simulink model "siglearmV7XYZforcecontrol"  (R2024b)
settings: Solver=VariableStepAuto  StartTime=0.0  StopTime=0.6  RelTol=1e-3
undefined symbols (not defined in the file): X, Y, Z
libraries: sm_lib x40, nesl_utility x40
(part 1 of 2)
settings Model: Creator=ChangZhiYuan  LastModifiedBy=20844
settings OptimizationCC: ReuseModelBlockBuffer=off
settings RTWCC: GPUComputeCapability=3.5

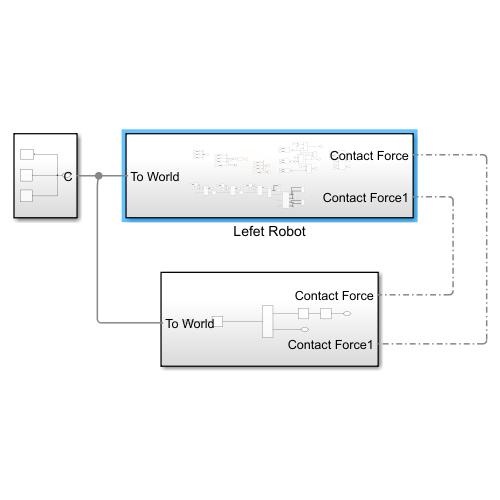
[thumbnail: Simulink's stored preview of the top-level diagram]
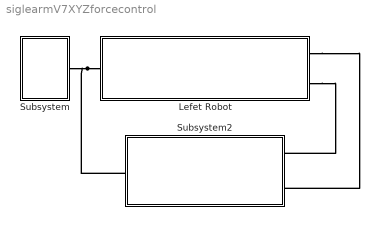
== system siglearmV7XYZforcecontrol ==
  Lefet Robot : Subsystem
  Subsystem : Subsystem
  Subsystem2 : Subsystem
  connections:
  Lefet Robot/LConn1 -- Subsystem2/LConn1 -- Subsystem/RConn1
  Lefet Robot/RConn2 -- Subsystem2/RConn1
  Lefet Robot/RConn1 -- Subsystem2/RConn2

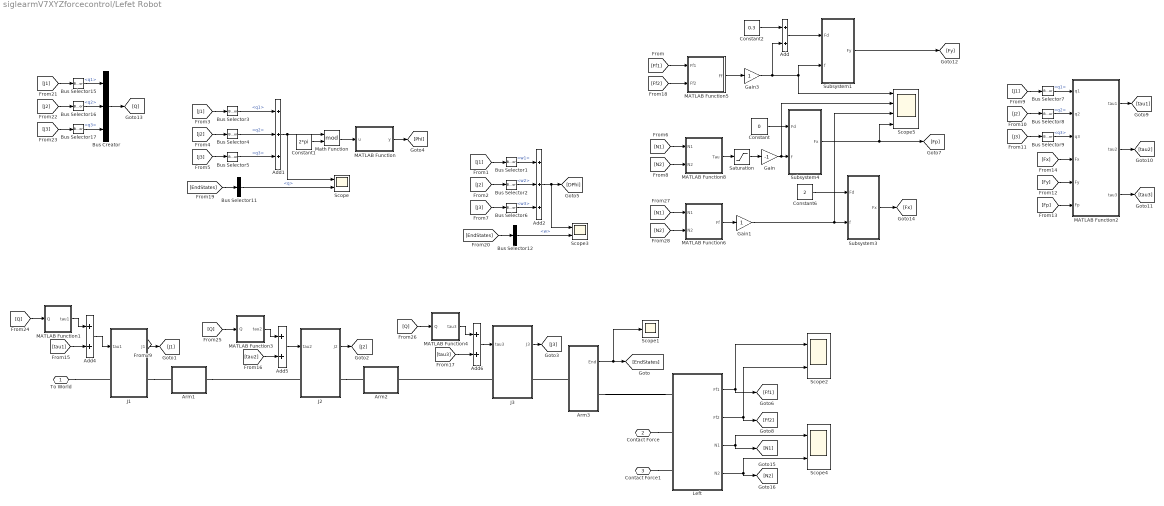
== system siglearmV7XYZforcecontrol/Lefet Robot ==
  Add{,4..6} (4 alike) : Sum
  Add1 : Sum  Inputs=+++
  Add2 : Sum  Inputs=+++
  Arm1 : Subsystem
  Arm2 : Subsystem
  Arm3 : Subsystem
  Bus Creator : BusCreator  Inputs=3
  Bus Selector1 : BusSelector  OutputSignals=w1
  Bus Selector11 : BusSelector  OutputSignals=q
  Bus Selector12 : BusSelector  OutputSignals=w
  Bus Selector15 : BusSelector  OutputSignals=q1
  Bus Selector16 : BusSelector  OutputSignals=q2
  Bus Selector17 : BusSelector  OutputSignals=q3
  Bus Selector2 : BusSelector  OutputSignals=w2
  Bus Selector3 : BusSelector  OutputSignals=q1
  Bus Selector4 : BusSelector  OutputSignals=q2
  Bus Selector5 : BusSelector  OutputSignals=q3
  Bus Selector6 : BusSelector  OutputSignals=w3
  Bus Selector7 : BusSelector  OutputSignals=q1
  Bus Selector8 : BusSelector  OutputSignals=q2
  Bus Selector9 : BusSelector  OutputSignals=q3
  Constant : Constant  Value=0
  Constant1 : Constant  Value=2*pi
  Constant2 : Constant  Value=0.3
  Constant6 : Constant  Value=2
  Gain : Gain  Gain=-1
  Gain1 : Gain
  Gain3 : Gain
  J1 : Subsystem
  J2 : Subsystem
  J3 : Subsystem
  Left : Subsystem
  MATLAB Function : MATLAB Function  TreatAsAtomicUnit=on
  MATLAB Function1 : MATLAB Function  TreatAsAtomicUnit=on
  MATLAB Function2 : MATLAB Function  TreatAsAtomicUnit=on
  MATLAB Function3 : MATLAB Function  TreatAsAtomicUnit=on
  MATLAB Function4 : MATLAB Function  TreatAsAtomicUnit=on
  MATLAB Function5 : MATLAB Function  TreatAsAtomicUnit=on
  MATLAB Function6 : MATLAB Function  TreatAsAtomicUnit=on
  MATLAB Function8 : MATLAB Function  TreatAsAtomicUnit=on
  Math Function : Math  Operator=mod
  Saturation : Saturate  UpperLimit=1  LowerLimit=-1
  Scope{,2..4} (4 alike) : Scope  NumInputPorts=2
  Scope1 : Scope
  Scope5 : Scope  NumInputPorts=4
  Subsystem1 : Subsystem
  Subsystem3 : Subsystem
  Subsystem4 : Subsystem
  To World : PMIOPort  Side=Left
  Contact Force : PMIOPort  Port=2  Side=Right
  Contact Force1 : PMIOPort  Port=3  Side=Right
  wires:
  Bus Selector9/1 -> MATLAB Function2/3(q3)  "<q3>"
  Add4/1 -> J1/1(tau1)
  Bus Selector7/1 -> MATLAB Function2/1(q1)  "<q1>"
  MATLAB Function2/1(tau1) -> [tau1]
  [EndStates] -> Bus Selector11/1
  [J2] -> Bus Selector4/1
  Bus Selector3/1 -> Add1/1  "<q1>"
  J2/1(J2) -> [J2]
  [J1] -> Bus Selector7/1
  [Fy] -> MATLAB Function2/5(Fy)
  Constant1/1 -> Math Function/2
  [J3] -> Bus Selector5/1
  Bus Selector2/1 -> Add2/2  "<w2>"
  [J1] -> Bus Selector1/1
  Bus Selector8/1 -> MATLAB Function2/2(q2)  "<q2>"
  Add1/1 -> Math Function/1, Scope/1
  Add6/1 -> J3/1(tau3)
  MATLAB Function2/2(tau2) -> [tau2]
  Math Function/1 -> MATLAB Function/1(u)
  Bus Selector12/1 -> Scope3/2  "<w>"
  [tau2] -> Add5/2
  Add2/1 -> Scope3/1, [DPhi]
  MATLAB Function2/3(tau3) -> [tau3]
  [J1] -> Bus Selector3/1
  [J3] -> Bus Selector9/1
  Bus Selector6/1 -> Add2/3  "<w3>"
  Bus Selector11/1 -> Scope/2  "<q>"
  [Fx] -> MATLAB Function2/4(Fx)
  Bus Selector4/1 -> Add1/2  "<q2>"
  Add5/1 -> J2/1(tau2)
  Bus Selector5/1 -> Add1/3  "<q3>"
  [J2] -> Bus Selector8/1
  J3/1(J3) -> [J3]
  J1/1(J1) -> [J1]
  [J3] -> Bus Selector6/1
  Bus Selector1/1 -> Add2/1  "<w1>"
  [EndStates] -> Bus Selector12/1
  [J2] -> Bus Selector2/1
  [Fp] -> MATLAB Function2/6(Fp)
  [tau1] -> Add4/2
  Subsystem4/1(Fx) -> Scope5/4, [Fp]
  Constant/1 -> Subsystem4/1(Fd)
  Arm3/1(End) -> Scope1/1, [EndStates]
  MATLAB Function/1(y) -> [Phi]
  Gain3/1 -> Add/2, Scope5/1, Subsystem1/2(f)
  [J2] -> Bus Selector16/1
  [J3] -> Bus Selector17/1
  [J1] -> Bus Selector15/1
  Bus Selector15/1 -> Bus Creator/1  "<q1>"
  Bus Selector16/1 -> Bus Creator/2  "<q2>"
  Bus Selector17/1 -> Bus Creator/3  "<q3>"
  Bus Creator/1 -> [Q]
  [Q] -> MATLAB Function1/1(Q)
  [Q] -> MATLAB Function3/1(Q)
  [tau3] -> Add6/2
  [Q] -> MATLAB Function4/1(Q)
  MATLAB Function1/1(tau1) -> Add4/1
  MATLAB Function3/1(tau2) -> Add5/1
  MATLAB Function4/1(tau3) -> Add6/1
  Constant6/1 -> Subsystem3/1(Fd)
  Subsystem3/1(Fx) -> [Fx]
  Subsystem1/1(Fy) -> [Fy]
  Constant2/1 -> Add/1
  Add/1 -> Subsystem1/1(Fd)
  Left/1(Ff1) -> [Ff1], Scope2/1
  Left/2(Ff2) -> [Ff2], Scope2/2
  Left/3(N1) -> [N1], Scope4/1
  Left/4(N2) -> [N2], Scope4/2
  [Ff1] -> MATLAB Function5/1(Ff1)
  [Ff2] -> MATLAB Function5/2(Ff2)
  MATLAB Function5/1(Ff) -> Gain3/1
  [N1] -> MATLAB Function6/1(N1)
  [N2] -> MATLAB Function6/2(N2)
  MATLAB Function6/1(Ff) -> Gain1/1
  Gain1/1 -> Scope5/3, Subsystem3/2(f)
  [N2] -> MATLAB Function8/2(N2)
  [N1] -> MATLAB Function8/1(N1)
  MATLAB Function8/1(Tau) -> Saturation/1
  Saturation/1 -> Gain/1
  Gain/1 -> Scope5/2, Subsystem4/2(f)
  connections:
  J1/RConn1 -- Arm1/LConn1
  Arm3/LConn1 -- J3/RConn1
  J3/LConn1 -- Arm2/RConn1
  J2/RConn1 -- Arm2/LConn1
  Left/LConn1 -- Arm3/RConn1
  Arm1/RConn1 -- J2/LConn1
  To World/RConn1 -- J1/LConn1
  Contact Force1/RConn1 -- Left/LConn3
  Contact Force/RConn1 -- Left/LConn2

== system siglearmV7XYZforcecontrol/Subsystem ==
  Mechanism Configuration : sm_lib/Utilities/Mechanism Configuration  UniformGravity=Constant  GravityVector=[0 -9.80665 0]  GravityVectorUnits=m/s^2  LinearizationDelta=0.001  JointModeTransitionNonlinearIterations=2
  Solver Configuration : nesl_utility/Solver Configuration  PhysicalDomain=network_engine_domain  SubClassName=solver  LeftPortType=input  RightPortType=generic  Tones=[]  Harmonics=[]  SimulateNoise=off  Profile=off  UseLocalSampling=off  EnableSwitchedLinearOptims=on  FrequencyDomain=off  UseCCode=off  RelTol=0.001  AbsTol=1e-06  MinStep=1e-09  ToWorkspace=off  RevertToSquareIcSolve=off  NumHomotopyIterations=100  PhasorMode=off  PhasorModeNumHarmonics=1  ConsistencySolver=NEWTON_FTOL  IndexReductionMethod=DerivativeReplacement  DoDC=off  ResidualTolerance=1e-09  ConsistencyTolSource=GLOBAL  ConsistencyAbsTol=0.001  ConsistencyRelTol=0.001  ConsistencyTolFactor=0.001  UseLocalSolver=off  LocalSolverChoice=NE_BACKWARD_EULER_ADVANCER  ResolveIndetEquations=on  FunctionEvalNumThread=1  LocalSolverSampleTime=0.001  DoFixedCost=off  MaxNonlinIter=3  MaxModeIter=2  ComputeImpulses=off  ImpulseIterations=2  LinearAlgebra=auto  LinearAlgebraNumThread=0  EquationFormulation=NE_TIME_EF  DelaysMemoryBudget=1024  AutomaticFiltering=on  FilteringTimeConstant=0.001  PartitionStorageMethod=AS_NEEDED  PartitionMemoryBudget=1024  PartitionMethod=ROBUST  MultibodyUseLocalSolver=off  MultibodyLocalSolverChoice=ODE1  MultibodyLocalSolverSampleTime=0.001
  World Frame : sm_lib/Frames and Transforms/World Frame
  C : PMIOPort  Side=Right
  connections:
  C/RConn1 -- Mechanism Configuration/RConn1 -- World Frame/RConn1 -- Solver Configuration/RConn1

== system siglearmV7XYZforcecontrol/Subsystem2 ==
  Object : sm_lib/Body Elements/Brick Solid  BrickDimensions=[0.01 1.5 0.5]  BrickDimensionsUnits=m  ExportEntireGeometry=on  InertiaType=CalculateFromGeometry  BasedOnType=Density  Density=100  DensityUnits=kg/m^3  Mass=1  MassUnits=kg  CenterOfMass=[0 0 0]  CenterOfMassUnits=m  MomentsOfInertia=[1 1 1]  MomentsOfInertiaUnits=kg*m^2  ProductsOfInertia=[0 0 0]  ProductsOfInertiaUnits=kg*m^2  GraphicType=FromGeometry  MarkerShape=Sphere  MarkerSize=10  GraphicVisPropType=SimpleVisualProperties  GraphicDiffuseColor=[0.5 0.5 0.5]  GraphicOpacity=1.0  GraphicSpecularColor=[0.5 0.5 0.5 1.0]  GraphicAmbientColor=[0.15 0.15 0.15 1.0]  GraphicEmissiveColor=[0.0 0.0 0.0 1.0]  GraphicShininess=75  DoExposeReferenceFrame=on  SerializedFrames=<Frames><Frame><Id>Frame1</Id><Value><Name>F1</Name><Origin><Source>GeometricFeature</Source><FeatureName>-x surface</FeatureName></Origin><PrimaryAxis><DefinedDirection>+Z</DefinedDirection><Source>ReferenceFrame</Source><SourceDirection>+Z</SourceDirection><FeatureName></FeatureName></PrimaryAxis><SecondaryAxis><DefinedDirection>+X</DefinedDirection><Source>ReferenceFrame</Source><SourceDirection>+X</SourceDirection><FeatureName></FeatureName></SecondaryAxis></Value></Frame></Frames>
  Revolved Solid : sm_lib/Body Elements/Revolved Solid  RevolutionCrossSection=[1 0.1; 1 -0.1; 1.01 -0.1; 1.01 0.1]  RevolutionCrossSectionUnits=m  RevolutionExtent=Custom  RevolutionAngle=30  RevolutionAngleUnits=deg  ExportConvexHullGeometry=on  InertiaType=CalculateFromGeometry  BasedOnType=Density  Density=1000  DensityUnits=kg/m^3  Mass=1  MassUnits=kg  CenterOfMass=[0 0 0]  CenterOfMassUnits=m  MomentsOfInertia=[1 1 1]  MomentsOfInertiaUnits=kg*m^2  ProductsOfInertia=[0 0 0]  ProductsOfInertiaUnits=kg*m^2  GraphicType=FromGeometry  MarkerShape=Sphere  MarkerSize=10  GraphicVisPropType=SimpleVisualProperties  GraphicDiffuseColor=[0.5 0.5 0.5]  GraphicOpacity=1.0  GraphicSpecularColor=[0.5 0.5 0.5 1.0]  GraphicAmbientColor=[0.15 0.15 0.15 1.0]  GraphicEmissiveColor=[0.0 0.0 0.0 1.0]  GraphicShininess=75  DoExposeReferenceFrame=on  SerializedFrames=<Frames/>
  Rigid Transform : sm_lib/Frames and Transforms/Rigid Transform  RotationMethod=None  FollAlignAxisA=+X  BaseAlignAxisA=+Y  FollAlignAxisB=+Y  BaseAlignAxisB=+Z  RotationStandardAxis=+Z  RotationAngle=0.0  RotationAngleUnits=deg  RotationArbitraryAxis=[0 0 1]  RotationSequenceAxes=FollowerAxes  RotationSequence=XYX  RotationSequenceAngles=[0 0 0]  RotationSequenceAnglesUnits=deg  RotationMatrix=[1 0 0; 0 1 0; 0 0 1]  Quaternion=[1 0 0 0]  TranslationMethod=Cartesian  TranslationCartesianOffset=[0.4505+0.005 0.5 0]  TranslationCartesianOffsetUnits=m  TranslationStandardAxis=+Z  TranslationStandardOffset=0  TranslationStandardOffsetUnits=m  TranslationROffset=0  TranslationROffsetUnits=m  TranslationThetaOffset=0  TranslationThetaOffsetUnits=deg  TranslationZOffset=0  TranslationZOffsetUnits=m
  Rigid Transform1 : sm_lib/Frames and Transforms/Rigid Transform  RotationMethod=StandardAxis  FollAlignAxisA=+X  BaseAlignAxisA=+Y  FollAlignAxisB=+Y  BaseAlignAxisB=+Z  RotationStandardAxis=+Z  RotationAngle=180  RotationAngleUnits=deg  RotationArbitraryAxis=[0 0 1]  RotationSequenceAxes=FollowerAxes  RotationSequence=XYX  RotationSequenceAngles=[0 0 0]  RotationSequenceAnglesUnits=deg  RotationMatrix=[1 0 0; 0 1 0; 0 0 1]  Quaternion=[1 0 0 0]  TranslationMethod=Cartesian  TranslationCartesianOffset=[0.98 0.1 0]  TranslationCartesianOffsetUnits=m  TranslationStandardAxis=+X  TranslationStandardOffset=0.98  TranslationStandardOffsetUnits=m  TranslationROffset=0  TranslationROffsetUnits=m  TranslationThetaOffset=0  TranslationThetaOffsetUnits=deg  TranslationZOffset=0  TranslationZOffsetUnits=m
  To World : PMIOPort  Side=Left
  Contact Force : PMIOPort  Port=2  Side=Right
  Contact Force1 : PMIOPort  Port=3  Side=Right
  connections:
  Rigid Transform/RConn1 -- Object/RConn1
  Rigid Transform/LConn1 -- To World/RConn1
  Object/LConn2 -- Contact Force/RConn1
  Rigid Transform1/LConn1 -- Object/LConn1
  Revolved Solid/RConn1 -- Rigid Transform1/RConn1
  Contact Force1/RConn1 -- Revolved Solid/LConn1

== system siglearmV7XYZforcecontrol/Lefet Robot/Arm1 ==
  Brick Solid : sm_lib/Body Elements/Brick Solid  BrickDimensions=[0.5 0.05 0.05]  BrickDimensionsUnits=m  ExportEntireGeometry=off  InertiaType=CalculateFromGeometry  BasedOnType=Density  Density=100  DensityUnits=kg/m^3  Mass=1  MassUnits=kg  CenterOfMass=[0 0 0]  CenterOfMassUnits=m  MomentsOfInertia=[1 1 1]  MomentsOfInertiaUnits=kg*m^2  ProductsOfInertia=[0 0 0]  ProductsOfInertiaUnits=kg*m^2  GraphicType=FromGeometry  MarkerShape=Sphere  MarkerSize=10  GraphicVisPropType=SimpleVisualProperties  GraphicDiffuseColor=[0.0 1.0 0.2]  GraphicOpacity=1.0  GraphicSpecularColor=[0.5 0.5 0.5 1.0]  GraphicAmbientColor=[0.15 0.15 0.15 1.0]  GraphicEmissiveColor=[0.0 0.0 0.0 1.0]  GraphicShininess=75  DoExposeReferenceFrame=on  SerializedFrames=<Frames><Frame><Id>Frame1</Id><Value><Name>F</Name><Origin><Source>CenterOfMassFrame</Source><FeatureName></FeatureName></Origin><PrimaryAxis><DefinedDirection>+Z</DefinedDirection><Source>ReferenceFrame</Source><SourceDirection>+Z</SourceDirection><FeatureName></FeatureName></PrimaryAxis><SecondaryAxis><DefinedDirection>+X</DefinedDirection><Source>ReferenceFrame</Source><SourceDirection>+X</SourceDirection><FeatureName></FeatureName></SecondaryAxis></Value></Frame></Frames>
  Cylindrical Solid : sm_lib/Body Elements/Cylindrical Solid  CylinderRadius=0.04  CylinderRadiusUnits=m  CylinderLength=0.06  CylinderLengthUnits=m  ExportEntireGeometry=off  InertiaType=CalculateFromGeometry  BasedOnType=Density  Density=1e-6  DensityUnits=kg/m^3  Mass=1  MassUnits=kg  CenterOfMass=[0 0 0]  CenterOfMassUnits=m  MomentsOfInertia=[1 1 1]  MomentsOfInertiaUnits=kg*m^2  ProductsOfInertia=[0 0 0]  ProductsOfInertiaUnits=kg*m^2  GraphicType=FromGeometry  MarkerShape=Sphere  MarkerSize=10  GraphicVisPropType=SimpleVisualProperties  GraphicDiffuseColor=[1.0 0.0 0.2]  GraphicOpacity=1.0  GraphicSpecularColor=[0.5 0.5 0.5 1.0]  GraphicAmbientColor=[0.15 0.15 0.15 1.0]  GraphicEmissiveColor=[0.0 0.0 0.0 1.0]  GraphicShininess=75  DoExposeReferenceFrame=on  SerializedFrames=<Frames><Frame><Id>Frame1</Id><Value><Name>F1</Name><Origin><Source>CenterOfMassFrame</Source><FeatureName></FeatureName></Origin><PrimaryAxis><DefinedDirection>+Z</DefinedDirection><Source>ReferenceFrame</Source><SourceDirection>+Z</SourceDirection><FeatureName></FeatureName></PrimaryAxis><SecondaryAxis><DefinedDirection>+X</DefinedDirection><Source>ReferenceFrame</Source><SourceDirection>+X</SourceDirection><FeatureName></FeatureName></SecondaryAxis></Value></Frame></Frames>
  Rigid Transform : sm_lib/Frames and Transforms/Rigid Transform  RotationMethod=None  FollAlignAxisA=+X  BaseAlignAxisA=+Y  FollAlignAxisB=+Y  BaseAlignAxisB=+Z  RotationStandardAxis=+Z  RotationAngle=0.0  RotationAngleUnits=deg  RotationArbitraryAxis=[0 0 1]  RotationSequenceAxes=FollowerAxes  RotationSequence=XYX  RotationSequenceAngles=[0 0 0]  RotationSequenceAnglesUnits=deg  RotationMatrix=[1 0 0; 0 1 0; 0 0 1]  Quaternion=[1 0 0 0]  TranslationMethod=StandardAxis  TranslationCartesianOffset=[0 0 0]  TranslationCartesianOffsetUnits=m  TranslationStandardAxis=+X  TranslationStandardOffset=0.25  TranslationStandardOffsetUnits=m  TranslationROffset=0  TranslationROffsetUnits=m  TranslationThetaOffset=0  TranslationThetaOffsetUnits=deg  TranslationZOffset=0  TranslationZOffsetUnits=m
  Rigid Transform1 : sm_lib/Frames and Transforms/Rigid Transform  RotationMethod=None  FollAlignAxisA=+X  BaseAlignAxisA=+Y  FollAlignAxisB=+Y  BaseAlignAxisB=+Z  RotationStandardAxis=+Z  RotationAngle=0.0  RotationAngleUnits=deg  RotationArbitraryAxis=[0 0 1]  RotationSequenceAxes=FollowerAxes  RotationSequence=XYX  RotationSequenceAngles=[0 0 0]  RotationSequenceAnglesUnits=deg  RotationMatrix=[1 0 0; 0 1 0; 0 0 1]  Quaternion=[1 0 0 0]  TranslationMethod=StandardAxis  TranslationCartesianOffset=[0 0 0]  TranslationCartesianOffsetUnits=m  TranslationStandardAxis=+X  TranslationStandardOffset=0.25  TranslationStandardOffsetUnits=m  TranslationROffset=0  TranslationROffsetUnits=m  TranslationThetaOffset=0  TranslationThetaOffsetUnits=deg  TranslationZOffset=0  TranslationZOffsetUnits=m
  To J1 : PMIOPort  Side=Left
  To J2 : PMIOPort  Port=2  Side=Right
  connections:
  Brick Solid/LConn1 -- Rigid Transform1/LConn1
  Rigid Transform/RConn1 -- Brick Solid/RConn1
  To J2/RConn1 -- Rigid Transform1/RConn1
  Cylindrical Solid/RConn1 -- To J1/RConn1
  Cylindrical Solid/LConn1 -- Rigid Transform/LConn1

== system siglearmV7XYZforcecontrol/Lefet Robot/Arm2 ==
  Brick Solid1 : sm_lib/Body Elements/Brick Solid  BrickDimensions=[0.5 0.05 0.05]  BrickDimensionsUnits=m  ExportEntireGeometry=off  InertiaType=CalculateFromGeometry  BasedOnType=Density  Density=100  DensityUnits=kg/m^3  Mass=1  MassUnits=kg  CenterOfMass=[0 0 0]  CenterOfMassUnits=m  MomentsOfInertia=[1 1 1]  MomentsOfInertiaUnits=kg*m^2  ProductsOfInertia=[0 0 0]  ProductsOfInertiaUnits=kg*m^2  GraphicType=FromGeometry  MarkerShape=Sphere  MarkerSize=10  GraphicVisPropType=SimpleVisualProperties  GraphicDiffuseColor=[0.2 1.0 0.0]  GraphicOpacity=1.0  GraphicSpecularColor=[0.5 0.5 0.5 1.0]  GraphicAmbientColor=[0.15 0.15 0.15 1.0]  GraphicEmissiveColor=[0.0 0.0 0.0 1.0]  GraphicShininess=75  DoExposeReferenceFrame=on  SerializedFrames=<Frames><Frame><Id>Frame1</Id><Value><Name>F</Name><Origin><Source>CenterOfMassFrame</Source><FeatureName></FeatureName></Origin><PrimaryAxis><DefinedDirection>+Z</DefinedDirection><Source>ReferenceFrame</Source><SourceDirection>+Z</SourceDirection><FeatureName></FeatureName></PrimaryAxis><SecondaryAxis><DefinedDirection>+X</DefinedDirection><Source>ReferenceFrame</Source><SourceDirection>+X</SourceDirection><FeatureName></FeatureName></SecondaryAxis></Value></Frame></Frames>
  Cylindrical Solid : sm_lib/Body Elements/Cylindrical Solid  CylinderRadius=0.04  CylinderRadiusUnits=m  CylinderLength=0.06  CylinderLengthUnits=m  ExportEntireGeometry=off  InertiaType=CalculateFromGeometry  BasedOnType=Density  Density=1e-6  DensityUnits=kg/m^3  Mass=1  MassUnits=kg  CenterOfMass=[0 0 0]  CenterOfMassUnits=m  MomentsOfInertia=[1 1 1]  MomentsOfInertiaUnits=kg*m^2  ProductsOfInertia=[0 0 0]  ProductsOfInertiaUnits=kg*m^2  GraphicType=FromGeometry  MarkerShape=Sphere  MarkerSize=10  GraphicVisPropType=SimpleVisualProperties  GraphicDiffuseColor=[1.0 0.0 0.2]  GraphicOpacity=1.0  GraphicSpecularColor=[0.5 0.5 0.5 1.0]  GraphicAmbientColor=[0.15 0.15 0.15 1.0]  GraphicEmissiveColor=[0.0 0.0 0.0 1.0]  GraphicShininess=75  DoExposeReferenceFrame=on  SerializedFrames=<Frames><Frame><Id>Frame1</Id><Value><Name>F1</Name><Origin><Source>CenterOfMassFrame</Source><FeatureName></FeatureName></Origin><PrimaryAxis><DefinedDirection>+Z</DefinedDirection><Source>ReferenceFrame</Source><SourceDirection>+Z</SourceDirection><FeatureName></FeatureName></PrimaryAxis><SecondaryAxis><DefinedDirection>+X</DefinedDirection><Source>ReferenceFrame</Source><SourceDirection>+X</SourceDirection><FeatureName></FeatureName></SecondaryAxis></Value></Frame></Frames>
  Rigid Transform2 : sm_lib/Frames and Transforms/Rigid Transform  RotationMethod=None  FollAlignAxisA=+X  BaseAlignAxisA=+Y  FollAlignAxisB=+Y  BaseAlignAxisB=+Z  RotationStandardAxis=+Z  RotationAngle=0.0  RotationAngleUnits=deg  RotationArbitraryAxis=[0 0 1]  RotationSequenceAxes=FollowerAxes  RotationSequence=XYX  RotationSequenceAngles=[0 0 0]  RotationSequenceAnglesUnits=deg  RotationMatrix=[1 0 0; 0 1 0; 0 0 1]  Quaternion=[1 0 0 0]  TranslationMethod=StandardAxis  TranslationCartesianOffset=[0 0 0]  TranslationCartesianOffsetUnits=m  TranslationStandardAxis=+X  TranslationStandardOffset=0.25  TranslationStandardOffsetUnits=m  TranslationROffset=0  TranslationROffsetUnits=m  TranslationThetaOffset=0  TranslationThetaOffsetUnits=deg  TranslationZOffset=0  TranslationZOffsetUnits=m
  Rigid Transform3 : sm_lib/Frames and Transforms/Rigid Transform  RotationMethod=None  FollAlignAxisA=+X  BaseAlignAxisA=+Y  FollAlignAxisB=+Y  BaseAlignAxisB=+Z  RotationStandardAxis=+Z  RotationAngle=0.0  RotationAngleUnits=deg  RotationArbitraryAxis=[0 0 1]  RotationSequenceAxes=FollowerAxes  RotationSequence=XYX  RotationSequenceAngles=[0 0 0]  RotationSequenceAnglesUnits=deg  RotationMatrix=[1 0 0; 0 1 0; 0 0 1]  Quaternion=[1 0 0 0]  TranslationMethod=StandardAxis  TranslationCartesianOffset=[0 0 0]  TranslationCartesianOffsetUnits=m  TranslationStandardAxis=+X  TranslationStandardOffset=0.25  TranslationStandardOffsetUnits=m  TranslationROffset=0  TranslationROffsetUnits=m  TranslationThetaOffset=0  TranslationThetaOffsetUnits=deg  TranslationZOffset=0  TranslationZOffsetUnits=m
  To J2 : PMIOPort  Side=Left
  To J3 : PMIOPort  Port=2  Side=Right
  connections:
  Rigid Transform2/RConn1 -- Brick Solid1/RConn1
  To J3/RConn1 -- Rigid Transform3/RConn1
  Brick Solid1/LConn1 -- Rigid Transform3/LConn1
  Cylindrical Solid/RConn1 -- To J2/RConn1
  Cylindrical Solid/LConn1 -- Rigid Transform2/LConn1

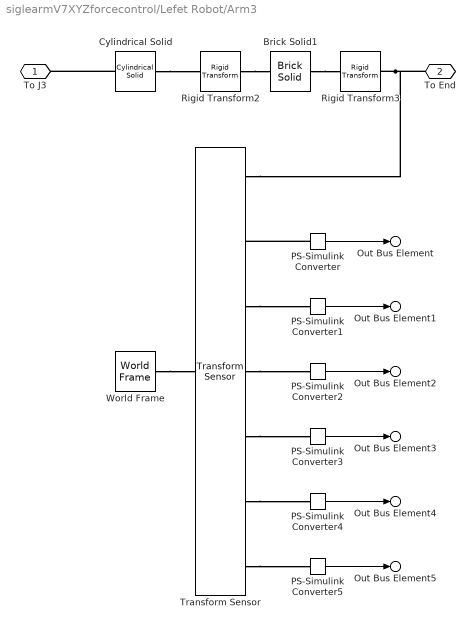
== system siglearmV7XYZforcecontrol/Lefet Robot/Arm3 ==
  Brick Solid1 : sm_lib/Body Elements/Brick Solid  BrickDimensions=[0.1 0.03 0.03]  BrickDimensionsUnits=m  ExportEntireGeometry=off  InertiaType=CalculateFromGeometry  BasedOnType=Density  Density=100  DensityUnits=kg/m^3  Mass=1  MassUnits=kg  CenterOfMass=[0 0 0]  CenterOfMassUnits=m  MomentsOfInertia=[1 1 1]  MomentsOfInertiaUnits=kg*m^2  ProductsOfInertia=[0 0 0]  ProductsOfInertiaUnits=kg*m^2  GraphicType=FromGeometry  MarkerShape=Sphere  MarkerSize=10  GraphicVisPropType=SimpleVisualProperties  GraphicDiffuseColor=[0.2 1.0 0.0]  GraphicOpacity=1.0  GraphicSpecularColor=[0.5 0.5 0.5 1.0]  GraphicAmbientColor=[0.15 0.15 0.15 1.0]  GraphicEmissiveColor=[0.0 0.0 0.0 1.0]  GraphicShininess=75  DoExposeReferenceFrame=on  SerializedFrames=<Frames><Frame><Id>Frame1</Id><Value><Name>F</Name><Origin><Source>CenterOfMassFrame</Source><FeatureName></FeatureName></Origin><PrimaryAxis><DefinedDirection>+Z</DefinedDirection><Source>ReferenceFrame</Source><SourceDirection>+Z</SourceDirection><FeatureName></FeatureName></PrimaryAxis><SecondaryAxis><DefinedDirection>+X</DefinedDirection><Source>ReferenceFrame</Source><SourceDirection>+X</SourceDirection><FeatureName></FeatureName></SecondaryAxis></Value></Frame></Frames>
  Cylindrical Solid : sm_lib/Body Elements/Cylindrical Solid  CylinderRadius=0.04  CylinderRadiusUnits=m  CylinderLength=0.06  CylinderLengthUnits=m  ExportEntireGeometry=off  InertiaType=CalculateFromGeometry  BasedOnType=Density  Density=1e-6  DensityUnits=kg/m^3  Mass=1  MassUnits=kg  CenterOfMass=[0 0 0]  CenterOfMassUnits=m  MomentsOfInertia=[1 1 1]  MomentsOfInertiaUnits=kg*m^2  ProductsOfInertia=[0 0 0]  ProductsOfInertiaUnits=kg*m^2  GraphicType=FromGeometry  MarkerShape=Sphere  MarkerSize=10  GraphicVisPropType=SimpleVisualProperties  GraphicDiffuseColor=[1.0 0.0 0.2]  GraphicOpacity=1.0  GraphicSpecularColor=[0.5 0.5 0.5 1.0]  GraphicAmbientColor=[0.15 0.15 0.15 1.0]  GraphicEmissiveColor=[0.0 0.0 0.0 1.0]  GraphicShininess=75  DoExposeReferenceFrame=on  SerializedFrames=<Frames><Frame><Id>Frame1</Id><Value><Name>F1</Name><Origin><Source>CenterOfMassFrame</Source><FeatureName></FeatureName></Origin><PrimaryAxis><DefinedDirection>+Z</DefinedDirection><Source>ReferenceFrame</Source><SourceDirection>+Z</SourceDirection><FeatureName></FeatureName></PrimaryAxis><SecondaryAxis><DefinedDirection>+X</DefinedDirection><Source>ReferenceFrame</Source><SourceDirection>+X</SourceDirection><FeatureName></FeatureName></SecondaryAxis></Value></Frame></Frames>
  PS-Simulink Converter{,1..5} (6 alike) : nesl_utility/PS-Simulink Converter  PhysicalDomain=network_engine_domain  SubClassName=ps_output  LeftPortType=input  RightPortType=output  PseudoPeriodic=off  Frequencies=[]  VectorFormat=inherit  Unit=inherit  AffineConversion=off
  Rigid Transform2 : sm_lib/Frames and Transforms/Rigid Transform  RotationMethod=None  FollAlignAxisA=+X  BaseAlignAxisA=+Y  FollAlignAxisB=+Y  BaseAlignAxisB=+Z  RotationStandardAxis=+Z  RotationAngle=0.0  RotationAngleUnits=deg  RotationArbitraryAxis=[0 0 1]  RotationSequenceAxes=FollowerAxes  RotationSequence=XYX  RotationSequenceAngles=[0 0 0]  RotationSequenceAnglesUnits=deg  RotationMatrix=[1 0 0; 0 1 0; 0 0 1]  Quaternion=[1 0 0 0]  TranslationMethod=StandardAxis  TranslationCartesianOffset=[0 0 0]  TranslationCartesianOffsetUnits=m  TranslationStandardAxis=+X  TranslationStandardOffset=0.05  TranslationStandardOffsetUnits=m  TranslationROffset=0  TranslationROffsetUnits=m  TranslationThetaOffset=0  TranslationThetaOffsetUnits=deg  TranslationZOffset=0  TranslationZOffsetUnits=m
  Rigid Transform3 : sm_lib/Frames and Transforms/Rigid Transform  RotationMethod=None  FollAlignAxisA=+X  BaseAlignAxisA=+Y  FollAlignAxisB=+Y  BaseAlignAxisB=+Z  RotationStandardAxis=+Z  RotationAngle=0.0  RotationAngleUnits=deg  RotationArbitraryAxis=[0 0 1]  RotationSequenceAxes=FollowerAxes  RotationSequence=XYX  RotationSequenceAngles=[0 0 0]  RotationSequenceAnglesUnits=deg  RotationMatrix=[1 0 0; 0 1 0; 0 0 1]  Quaternion=[1 0 0 0]  TranslationMethod=StandardAxis  TranslationCartesianOffset=[0 0 0]  TranslationCartesianOffsetUnits=m  TranslationStandardAxis=+X  TranslationStandardOffset=0.05  TranslationStandardOffsetUnits=m  TranslationROffset=0  TranslationROffsetUnits=m  TranslationThetaOffset=0  TranslationThetaOffsetUnits=deg  TranslationZOffset=0  TranslationZOffsetUnits=m
  Transform Sensor : sm_lib/Frames and Transforms/Transform Sensor  MeasurementFrame=World  RotationSequence=XYX  SenseAngle=on  SenseAxis=off  SenseQ=off  SenseR=off  SenseRotationSequence=off  SenseOmegaX=off  SenseOmegaY=off  SenseOmegaZ=on  SenseOmega=off  SenseQDot=off  SenseRDot=off  SenseRotationSequenceDot=off  SenseAlphaX=off  SenseAlphaY=off  SenseAlphaZ=off  SenseAlpha=off  SenseQDDot=off  SenseRDDot=off  SenseX=on  SenseY=on  SenseZ=off  SenseXYZ=off  SenseRad=off  SenseAzim=off  SenseDist=off  SenseInc=off  SenseXDot=on  SenseYDot=on  SenseZDot=off  SenseXYZDot=off  SenseRadDot=off  SenseAzimDot=off  SenseDistDot=off  SenseIncDot=off  SenseXDDot=off  SenseYDDot=off  SenseZDDot=off  SenseXYZDDot=off  SenseRadDDot=off  SenseAzimDDot=off  SenseDistDDot=off  SenseIncDDot=off
  World Frame : sm_lib/Frames and Transforms/World Frame
  To J3 : PMIOPort  Side=Left
  To End : PMIOPort  Port=2  Side=Right
  Out Bus Element : Outport  PortName=End  Element=q
  Out Bus Element1 : Outport  PortName=End  Element=w
  Out Bus Element2 : Outport  PortName=End  Element=x
  Out Bus Element3 : Outport  PortName=End  Element=y
  Out Bus Element4 : Outport  PortName=End  Element=vx
  Out Bus Element5 : Outport  PortName=End  Element=vy
  wires:
  PS-Simulink Converter/1 -> Out Bus Element/1
  PS-Simulink Converter1/1 -> Out Bus Element1/1
  PS-Simulink Converter2/1 -> Out Bus Element2/1
  PS-Simulink Converter5/1 -> Out Bus Element5/1
  PS-Simulink Converter4/1 -> Out Bus Element4/1
  PS-Simulink Converter3/1 -> Out Bus Element3/1
  connections:
  Rigid Transform2/RConn1 -- Brick Solid1/RConn1
  Rigid Transform3/RConn1 -- To End/RConn1 -- Transform Sensor/RConn1
  Brick Solid1/LConn1 -- Rigid Transform3/LConn1
  Cylindrical Solid/RConn1 -- To J3/RConn1
  Cylindrical Solid/LConn1 -- Rigid Transform2/LConn1
  World Frame/RConn1 -- Transform Sensor/LConn1
  PS-Simulink Converter/LConn1 -- Transform Sensor/RConn2
  Transform Sensor/RConn3 -- PS-Simulink Converter1/LConn1
  Transform Sensor/RConn5 -- PS-Simulink Converter3/LConn1
  Transform Sensor/RConn4 -- PS-Simulink Converter2/LConn1
  Transform Sensor/RConn7 -- PS-Simulink Converter5/LConn1
  Transform Sensor/RConn6 -- PS-Simulink Converter4/LConn1

== system siglearmV7XYZforcecontrol/Lefet Robot/J1 ==
  tau1 : Inport
  Constant : Constant  Value=2*pi
  Math Function : Math  Operator=mod
  PS-Simulink Converter4 : nesl_utility/PS-Simulink Converter  PhysicalDomain=network_engine_domain  SubClassName=ps_output  LeftPortType=input  RightPortType=output  PseudoPeriodic=off  Frequencies=[]  VectorFormat=inherit  Unit=inherit  AffineConversion=off
  PS-Simulink Converter5 : nesl_utility/PS-Simulink Converter  PhysicalDomain=network_engine_domain  SubClassName=ps_output  LeftPortType=input  RightPortType=output  PseudoPeriodic=off  Frequencies=[]  VectorFormat=inherit  Unit=inherit  AffineConversion=off
  Revolute Joint3 : sm_lib/Joints/Revolute Joint  JointMode=Normal  CompositeWrenchDir=FollowerOnBase  CompositeWrenchFrame=BaseFrame  SenseConstraintForce=off  SenseConstraintTorque=off  SenseTotalForce=off  SenseTotalTorque=off  PositionTargetSpecify=on  PositionTargetPriority=High  PositionTargetValue=1.7464  PositionTargetValueUnits=rad  VelocityTargetSpecify=off  VelocityTargetPriority=High  VelocityTargetValue=0  VelocityTargetValueUnits=deg/s  EquilibriumPosition=0  EquilibriumPositionUnits=deg  SpringStiffness=0  SpringStiffnessUnits=N*m/deg  DampingCoefficient=0  DampingCoefficientUnits=N*m/(deg/s)  LowerLimitSpecify=off  LowerLimitBound=-90  LowerLimitBoundUnits=deg  LowerLimitStiffness=1e4  LowerLimitStiffnessUnits=N*m/deg  LowerLimitDamping=10  LowerLimitDampingUnits=N*m/(deg/s)  LowerLimitTransitionRegionWidth=0.1  LowerLimitTransitionRegionWidthUnits=deg  UpperLimitSpecify=off  UpperLimitBound=90  UpperLimitBoundUnits=deg  UpperLimitStiffness=1e4  UpperLimitStiffnessUnits=N*m/deg  UpperLimitDamping=10  UpperLimitDampingUnits=N*m/(deg/s)  UpperLimitTransitionRegionWidth=0.1  UpperLimitTransitionRegionWidthUnits=deg  TorqueActuationMode=InputTorque  MotionActuationMode=ComputedMotion  SensePosition=on  SenseVelocity=on  SenseAcceleration=off  SenseTorqueForce=off  SenseLowerLimitTorqueForce=off  SenseUpperLimitTorqueForce=off
  Simulink-PS Converter : nesl_utility/Simulink-PS Converter  PhysicalDomain=network_engine_domain  SubClassName=ps_input  LeftPortType=input  RightPortType=output  PseudoPeriodic=off  Frequencies=[]  NoiseDistribution=none  NoiseParameters=[]  Unit=1  AffineConversion=off  FilteringAndDerivatives=provide  SimscapeFilterOrder=1  InputFilterTimeConstant=0.001  UdotUserProvided=0
  Conn1 : PMIOPort  Side=Right
  Conn2 : PMIOPort  Port=2  Side=Left
  Bus Element Out : Outport  PortName=J1  Element=q1
  Bus Element Out1 : Outport  PortName=J1  Element=w1
  wires:
  tau1/1 -> Simulink-PS Converter/1
  PS-Simulink Converter5/1 -> Bus Element Out1/1
  PS-Simulink Converter4/1 -> Bus Element Out/1, Math Function/1
  Constant/1 -> Math Function/2
  connections:
  Revolute Joint3/LConn2 -- Simulink-PS Converter/RConn1
  Revolute Joint3/RConn2 -- PS-Simulink Converter4/LConn1
  Revolute Joint3/RConn3 -- PS-Simulink Converter5/LConn1
  Revolute Joint3/RConn1 -- Conn1/RConn1
  Conn2/RConn1 -- Revolute Joint3/LConn1

== system siglearmV7XYZforcecontrol/Lefet Robot/J2 ==
  tau2 : Inport
  Constant : Constant  Value=2*pi
  Math Function : Math  Operator=mod
  PS-Simulink Converter2 : nesl_utility/PS-Simulink Converter  PhysicalDomain=network_engine_domain  SubClassName=ps_output  LeftPortType=input  RightPortType=output  PseudoPeriodic=off  Frequencies=[]  VectorFormat=inherit  Unit=inherit  AffineConversion=off
  PS-Simulink Converter3 : nesl_utility/PS-Simulink Converter  PhysicalDomain=network_engine_domain  SubClassName=ps_output  LeftPortType=input  RightPortType=output  PseudoPeriodic=off  Frequencies=[]  VectorFormat=inherit  Unit=inherit  AffineConversion=off
  Revolute Joint1 : sm_lib/Joints/Revolute Joint  JointMode=Normal  CompositeWrenchDir=FollowerOnBase  CompositeWrenchFrame=BaseFrame  SenseConstraintForce=off  SenseConstraintTorque=off  SenseTotalForce=off  SenseTotalTorque=off  PositionTargetSpecify=on  PositionTargetPriority=High  PositionTargetValue=-2.2523  PositionTargetValueUnits=rad  VelocityTargetSpecify=off  VelocityTargetPriority=High  VelocityTargetValue=0  VelocityTargetValueUnits=deg/s  EquilibriumPosition=0  EquilibriumPositionUnits=deg  SpringStiffness=0  SpringStiffnessUnits=N*m/deg  DampingCoefficient=0  DampingCoefficientUnits=N*m/(deg/s)  LowerLimitSpecify=off  LowerLimitBound=-90  LowerLimitBoundUnits=deg  LowerLimitStiffness=1e4  LowerLimitStiffnessUnits=N*m/deg  LowerLimitDamping=10  LowerLimitDampingUnits=N*m/(deg/s)  LowerLimitTransitionRegionWidth=0.1  LowerLimitTransitionRegionWidthUnits=deg  UpperLimitSpecify=off  UpperLimitBound=90  UpperLimitBoundUnits=deg  UpperLimitStiffness=1e4  UpperLimitStiffnessUnits=N*m/deg  UpperLimitDamping=10  UpperLimitDampingUnits=N*m/(deg/s)  UpperLimitTransitionRegionWidth=0.1  UpperLimitTransitionRegionWidthUnits=deg  TorqueActuationMode=InputTorque  MotionActuationMode=ComputedMotion  SensePosition=on  SenseVelocity=on  SenseAcceleration=off  SenseTorqueForce=off  SenseLowerLimitTorqueForce=off  SenseUpperLimitTorqueForce=off
  Simulink-PS Converter : nesl_utility/Simulink-PS Converter  PhysicalDomain=network_engine_domain  SubClassName=ps_input  LeftPortType=input  RightPortType=output  PseudoPeriodic=off  Frequencies=[]  NoiseDistribution=none  NoiseParameters=[]  Unit=1  AffineConversion=off  FilteringAndDerivatives=provide  SimscapeFilterOrder=1  InputFilterTimeConstant=0.001  UdotUserProvided=0
  Conn1 : PMIOPort  Side=Left
  Conn2 : PMIOPort  Port=2  Side=Right
  Bus Element Out : Outport  PortName=J2  Element=q2
  Bus Element Out1 : Outport  PortName=J2  Element=w2
  wires:
  tau2/1 -> Simulink-PS Converter/1
  PS-Simulink Converter3/1 -> Bus Element Out1/1
  Constant/1 -> Math Function/2
  PS-Simulink Converter2/1 -> Bus Element Out/1
  connections:
  Revolute Joint1/RConn3 -- PS-Simulink Converter3/LConn1
  Revolute Joint1/RConn2 -- PS-Simulink Converter2/LConn1
  Simulink-PS Converter/RConn1 -- Revolute Joint1/LConn2
  Revolute Joint1/RConn1 -- Conn2/RConn1
  Conn1/RConn1 -- Revolute Joint1/LConn1

== system siglearmV7XYZforcecontrol/Lefet Robot/J3 ==
  tau3 : Inport
  Constant : Constant  Value=2*pi
  Math Function : Math  Operator=mod
  PS-Simulink Converter : nesl_utility/PS-Simulink Converter  PhysicalDomain=network_engine_domain  SubClassName=ps_output  LeftPortType=input  RightPortType=output  PseudoPeriodic=off  Frequencies=[]  VectorFormat=inherit  Unit=inherit  AffineConversion=off
  PS-Simulink Converter1 : nesl_utility/PS-Simulink Converter  PhysicalDomain=network_engine_domain  SubClassName=ps_output  LeftPortType=input  RightPortType=output  PseudoPeriodic=off  Frequencies=[]  VectorFormat=inherit  Unit=inherit  AffineConversion=off
  Revolute Joint2 : sm_lib/Joints/Revolute Joint  JointMode=Normal  CompositeWrenchDir=FollowerOnBase  CompositeWrenchFrame=BaseFrame  SenseConstraintForce=off  SenseConstraintTorque=off  SenseTotalForce=off  SenseTotalTorque=off  PositionTargetSpecify=on  PositionTargetPriority=High  PositionTargetValue=0.5059  PositionTargetValueUnits=rad  VelocityTargetSpecify=off  VelocityTargetPriority=High  VelocityTargetValue=0  VelocityTargetValueUnits=deg/s  EquilibriumPosition=0  EquilibriumPositionUnits=deg  SpringStiffness=0  SpringStiffnessUnits=N*m/deg  DampingCoefficient=0  DampingCoefficientUnits=N*m/(deg/s)  LowerLimitSpecify=off  LowerLimitBound=-90  LowerLimitBoundUnits=deg  LowerLimitStiffness=1e4  LowerLimitStiffnessUnits=N*m/deg  LowerLimitDamping=10  LowerLimitDampingUnits=N*m/(deg/s)  LowerLimitTransitionRegionWidth=0.1  LowerLimitTransitionRegionWidthUnits=deg  UpperLimitSpecify=off  UpperLimitBound=90  UpperLimitBoundUnits=deg  UpperLimitStiffness=1e4  UpperLimitStiffnessUnits=N*m/deg  UpperLimitDamping=10  UpperLimitDampingUnits=N*m/(deg/s)  UpperLimitTransitionRegionWidth=0.1  UpperLimitTransitionRegionWidthUnits=deg  TorqueActuationMode=InputTorque  MotionActuationMode=ComputedMotion  SensePosition=on  SenseVelocity=on  SenseAcceleration=off  SenseTorqueForce=off  SenseLowerLimitTorqueForce=off  SenseUpperLimitTorqueForce=off
  Simulink-PS Converter1 : nesl_utility/Simulink-PS Converter  PhysicalDomain=network_engine_domain  SubClassName=ps_input  LeftPortType=input  RightPortType=output  PseudoPeriodic=off  Frequencies=[]  NoiseDistribution=none  NoiseParameters=[]  Unit=1  AffineConversion=off  FilteringAndDerivatives=provide  SimscapeFilterOrder=1  InputFilterTimeConstant=0.001  UdotUserProvided=0
  Conn1 : PMIOPort  Side=Left
  Conn2 : PMIOPort  Port=2  Side=Right
  Bus Element Out : Outport  PortName=J3  Element=q3
  Bus Element Out1 : Outport  PortName=J3  Element=w3
  wires:
  tau3/1 -> Simulink-PS Converter1/1
  PS-Simulink Converter1/1 -> Bus Element Out1/1
  Constant/1 -> Math Function/2
  PS-Simulink Converter/1 -> Bus Element Out/1
  connections:
  PS-Simulink Converter/LConn1 -- Revolute Joint2/RConn2
  Revolute Joint2/RConn3 -- PS-Simulink Converter1/LConn1
  Conn2/RConn1 -- Revolute Joint2/RConn1
  Revolute Joint2/LConn2 -- Simulink-PS Converter1/RConn1
  Revolute Joint2/LConn1 -- Conn1/RConn1

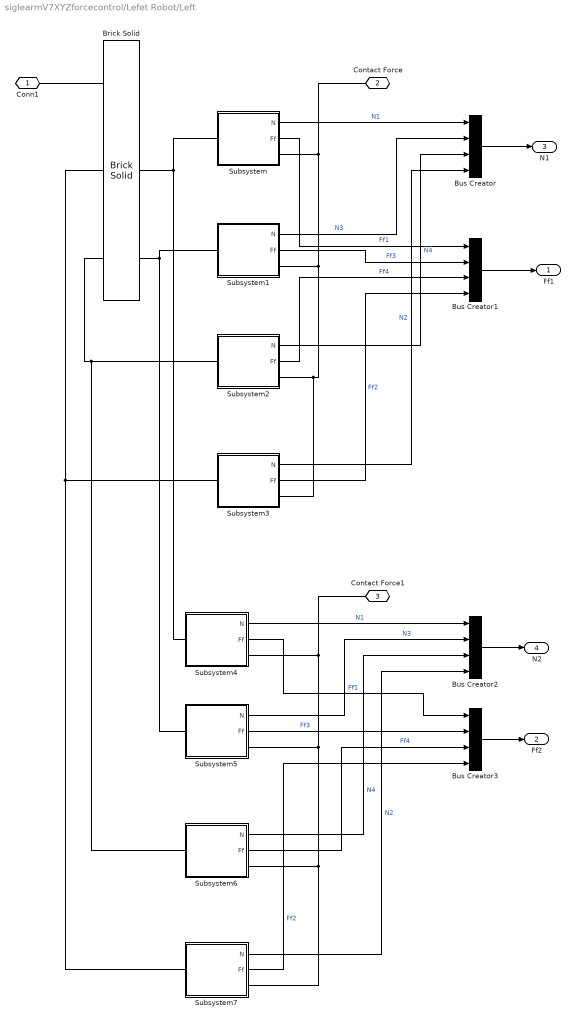
== system siglearmV7XYZforcecontrol/Lefet Robot/Left ==
  Brick Solid : sm_lib/Body Elements/Brick Solid  BrickDimensions=[0.001 0.04 0.04]  BrickDimensionsUnits=m  ExportEntireGeometry=off  InertiaType=CalculateFromGeometry  BasedOnType=Density  Density=1e-6  DensityUnits=kg/m^3  Mass=1  MassUnits=kg  CenterOfMass=[0 0 0]  CenterOfMassUnits=m  MomentsOfInertia=[1 1 1]  MomentsOfInertiaUnits=kg*m^2  ProductsOfInertia=[0 0 0]  ProductsOfInertiaUnits=kg*m^2  GraphicType=FromGeometry  MarkerShape=Sphere  MarkerSize=10  GraphicVisPropType=SimpleVisualProperties  GraphicDiffuseColor=[1.0 0.0 0.0]  GraphicOpacity=1.0  GraphicSpecularColor=[0.5 0.5 0.5 1.0]  GraphicAmbientColor=[0.15 0.15 0.15 1.0]  GraphicEmissiveColor=[0.0 0.0 0.0 1.0]  GraphicShininess=75  DoExposeReferenceFrame=on  SerializedFrames=<Frames><Frame><Id>Frame1</Id><Value><Name>F</Name><Origin><Source>GeometricFeature</Source><FeatureName>+x surface</FeatureName></Origin><PrimaryAxis><DefinedDirection>+Z</DefinedDirection><Source>ReferenceFrame</Source><SourceDirection>+Z</SourceDirection><FeatureName></FeatureName></PrimaryAxis><SecondaryAxis><DefinedDirection>+X</DefinedDirection><Source>ReferenceFrame</Source><SourceDirection>+X</SourceDirection><FeatureName></FeatureName></SecondaryAxis></Value></Frame><Frame><Id>Frame2</Id><Value><Name>F1</Name><Origin><Source>GeometricFeature</Source><FeatureName>+x +y +z point</FeatureName></Origin><PrimaryAxis><DefinedDirection>+Z</DefinedDirection><Source>ReferenceFrame</Source><SourceDirection>+Z</SourceDirection><FeatureName></FeatureName></PrimaryAxis><SecondaryAxis><DefinedDirection>+X</DefinedDirection><Source>ReferenceFrame</Source><SourceDirection>+X</SourceDirection><FeatureName></FeatureName></SecondaryAxis></Value></Frame><Frame><Id>Frame3</Id><Value><Name>F2</Name><Origin><Source>GeometricFeature</Source><FeatureName>+x -y +z point</FeatureName></Origin><PrimaryAxis><DefinedDirection>+Z</DefinedDirection><Source>ReferenceFrame</Source><SourceDirection>+Z</SourceDirection><FeatureName></FeatureName></PrimaryAxis><SecondaryAxis><DefinedDirection>+X</DefinedDirection><Source>ReferenceFrame</Source><SourceDirection>+X</SourceDirection><FeatureName></FeatureName></SecondaryAxis></Value></Frame><Frame><Id>Frame4</Id><Value><Name>F3</Name><Origin><Source>GeometricFeature</Source><FeatureName>+x -y -z point</FeatureName></Origin><PrimaryAxis><DefinedDirection>+Z</DefinedDirection><Source>ReferenceFrame</Source><SourceDirection>+Z</SourceDirection><FeatureName></FeatureName></PrimaryAxis><SecondaryAxis><DefinedDirection>+X</DefinedDirection><Source>ReferenceFrame</Source><SourceDirection>+X</SourceDirection><FeatureName></FeatureName></SecondaryAxis></Value></Frame><Frame><Id>Frame5</Id><Value><Name>F4</Name><Origin><Source>GeometricFeature</Source><FeatureName>+x +y -z point</FeatureName></Origin><PrimaryAxis><DefinedDirection>+Z</DefinedDirection><Source>ReferenceFrame</Source><SourceDirection>+Z</SourceDirection><FeatureName></FeatureName></PrimaryAxis><SecondaryAxis><DefinedDirection>+X</DefinedDirection><Source>ReferenceFrame</Source><SourceDirection>+X</SourceDirection><FeatureName></FeatureName></SecondaryAxis></Value></Frame></Frames>
  Bus Creator{,1..3} (4 alike) : BusCreator  Inputs=4
  Subsystem : Subsystem
  Subsystem1 : Subsystem
  Subsystem2 : Subsystem
  Subsystem3 : Subsystem
  Subsystem4 : Subsystem
  Subsystem5 : Subsystem
  Subsystem6 : Subsystem
  Subsystem7 : Subsystem
  Conn1 : PMIOPort  Side=Left
  Contact Force : PMIOPort  Port=2  Side=Left
  Contact Force1 : PMIOPort  Port=3  Side=Left
  Ff1 : Outport
  Ff2 : Outport  Port=2
  N1 : Outport  Port=3
  N2 : Outport  Port=4
  wires:
  Subsystem1/1(N) -> Bus Creator/2  "N3"
  Subsystem2/1(N) -> Bus Creator/3  "N4"
  Subsystem3/1(N) -> Bus Creator/4  "N2"
  Bus Creator1/1 -> Ff1/1
  Subsystem1/2(Ff) -> Bus Creator1/2  "Ff3"
  Subsystem2/2(Ff) -> Bus Creator1/3  "Ff4"
  Subsystem3/2(Ff) -> Bus Creator1/4  "Ff2"
  Subsystem4/2(Ff) -> Bus Creator3/1  "Ff1"
  Subsystem6/2(Ff) -> Bus Creator3/3  "Ff4"
  Subsystem5/2(Ff) -> Bus Creator3/2  "Ff3"
  Subsystem5/1(N) -> Bus Creator2/2  "N3"
  Subsystem7/2(Ff) -> Bus Creator3/4  "Ff2"
  Subsystem6/1(N) -> Bus Creator2/3  "N4"
  Subsystem7/1(N) -> Bus Creator2/4  "N2"
  Subsystem4/1(N) -> Bus Creator2/1  "N1"
  Bus Creator3/1 -> Ff2/1
  Subsystem/1(N) -> Bus Creator/1  "N1"
  Subsystem/2(Ff) -> Bus Creator1/1  "Ff1"
  Bus Creator/1 -> N1/1
  Bus Creator2/1 -> N2/1
  connections:
  Brick Solid/RConn1 -- Conn1/RConn1
  Subsystem1/LConn1 -- Subsystem5/LConn1 -- Brick Solid/LConn3
  Brick Solid/RConn3 -- Subsystem6/LConn1 -- Subsystem2/LConn1
  Brick Solid/RConn2 -- Subsystem7/LConn1 -- Subsystem3/LConn1
  Subsystem3/RConn1 -- Subsystem2/RConn1 -- Contact Force/RConn1 -- Subsystem/RConn1 -- Subsystem1/RConn1
  Contact Force1/RConn1 -- Subsystem7/RConn1 -- Subsystem6/RConn1 -- Subsystem5/RConn1 -- Subsystem4/RConn1
  Brick Solid/LConn2 -- Subsystem4/LConn1 -- Subsystem/LConn1

== system siglearmV7XYZforcecontrol/Lefet Robot/Subsystem1 ==
  Fd : Inport
  f : Inport  Port=2
  Constant2 : Constant  Value=200
  Constant4 : Constant  Value=20
  Constant6 : Constant  Value=200
  Constant7 : Constant  Value=20
  Control Y Position1 : Subsystem
  Scope : Scope  NumInputPorts=4
  TD : Subsystem
  TD1 : Subsystem
  Fy : Outport
  wires:
  TD1/2(V) -> Scope/4, Control Y Position1/4(vf)
  Constant2/1 -> TD/2(r)
  Constant6/1 -> TD1/2(r)
  f/1 -> TD1/1(Ref)
  Constant4/1 -> TD/3(xi)
  Constant7/1 -> TD1/3(xi)
  TD/1(P) -> Scope/1, Control Y Position1/1(Fd)
  TD/2(V) -> Scope/2, Control Y Position1/2(vFd)
  TD1/1(P) -> Scope/3, Control Y Position1/3(f)
  Control Y Position1/1(Fy) -> Fy/1
  Fd/1 -> TD/1(Ref)

== system siglearmV7XYZforcecontrol/Lefet Robot/Subsystem3 ==
  Fd : Inport
  f : Inport  Port=2
  Constant2 : Constant  Value=200
  Constant4 : Constant  Value=20
  Constant6 : Constant  Value=200
  Constant7 : Constant  Value=20
  Control Y Position1 : Subsystem
  Scope : Scope  NumInputPorts=4
  TD : Subsystem
  TD1 : Subsystem
  Fx : Outport
  wires:
  TD1/2(V) -> Scope/4, Control Y Position1/4(vf)
  Constant2/1 -> TD/2(r)
  Constant6/1 -> TD1/2(r)
  f/1 -> TD1/1(Ref)
  Constant4/1 -> TD/3(xi)
  Constant7/1 -> TD1/3(xi)
  TD/1(P) -> Scope/1, Control Y Position1/1(Fd)
  TD/2(V) -> Scope/2, Control Y Position1/2(vFd)
  TD1/1(P) -> Scope/3, Control Y Position1/3(f)
  Control Y Position1/1(Fy) -> Fx/1
  Fd/1 -> TD/1(Ref)

== system siglearmV7XYZforcecontrol/Lefet Robot/Subsystem4 ==
  Fd : Inport
  f : Inport  Port=2
  Constant2 : Constant  Value=200
  Constant4 : Constant  Value=20
  Constant6 : Constant  Value=200
  Constant7 : Constant  Value=20
  Control Y Position1 : Subsystem
  Scope : Scope  NumInputPorts=4
  Scope1 : Scope
  TD : Subsystem
  TD1 : Subsystem
  Fx : Outport
  wires:
  TD1/2(V) -> Scope/4, Control Y Position1/4(vf)
  Constant2/1 -> TD/2(r)
  Constant6/1 -> TD1/2(r)
  f/1 -> TD1/1(Ref)
  Constant4/1 -> TD/3(xi)
  Constant7/1 -> TD1/3(xi)
  TD/1(P) -> Control Y Position1/1(Fd), Scope/1
  TD/2(V) -> Control Y Position1/2(vFd), Scope/2
  TD1/1(P) -> Scope/3, Control Y Position1/3(f)
  Control Y Position1/1(Fy) -> Scope1/1, Fx/1
  Fd/1 -> TD/1(Ref)

== system siglearmV7XYZforcecontrol/Lefet Robot/Left/Subsystem ==
  PS-Simulink Converter1 : nesl_utility/PS-Simulink Converter  PhysicalDomain=network_engine_domain  SubClassName=ps_output  LeftPortType=input  RightPortType=output  PseudoPeriodic=off  Frequencies=[]  VectorFormat=inherit  Unit=inherit  AffineConversion=off
  PS-Simulink Converter2 : nesl_utility/PS-Simulink Converter  PhysicalDomain=network_engine_domain  SubClassName=ps_output  LeftPortType=input  RightPortType=output  PseudoPeriodic=off  Frequencies=[]  VectorFormat=inherit  Unit=inherit  AffineConversion=off
  PS-Simulink Converter4 : nesl_utility/PS-Simulink Converter  PhysicalDomain=network_engine_domain  SubClassName=ps_output  LeftPortType=input  RightPortType=output  PseudoPeriodic=off  Frequencies=[]  VectorFormat=inherit  Unit=inherit  AffineConversion=off
  Point : sm_lib/Curves and Surfaces/Point  GraphicType=None  MarkerShape=Sphere  MarkerSize=10  GraphicVisPropType=SimpleVisualProperties  GraphicDiffuseColor=[0.5 0.5 0.5]  GraphicOpacity=1.0  GraphicSpecularColor=[0.5 0.5 0.5 1.0]  GraphicAmbientColor=[0.15 0.15 0.15 1.0]  GraphicEmissiveColor=[0.0 0.0 0.0 1.0]  GraphicShininess=75
  Product : Product
  Product1 : Product
  Spatial Contact Force : sm_lib/Forces and Torques/Spatial Contact Force  NormalForceType=SmoothSpringDamper  NormalStiffness=1e6  NormalStiffnessUnits=N/m  NormalDamping=1e3  NormalDampingUnits=N/(m/s)  NormalTransitionRegionWidth=1e-3  NormalTransitionRegionWidthUnits=m  FrictionType=SmoothStickSlip  CoefficientOfStaticFriction=0.5  CoefficientOfDynamicFriction=0.3  FrictionalCriticalVelocity=1e-3  FrictionalCriticalVelocityUnits=m/s  SenseContactSignal=on  SensePenetrationDepth=off  SenseSeparationDistance=off  SenseNormalForceMagnitude=on  SenseFrictionalForceMagnitude=on  SenseNormalVelocity=off  SenseTangentialVelocity=off  SenseContactBaseRotation=off  SenseContactBaseTranslation=off  SenseContactFollowerRotation=off  SenseContactFollowerTranslation=off  ZeroCrossDetectContactStartAndEnd=off
  Conn1 : PMIOPort  Side=Right
  Conn2 : PMIOPort  Port=2  Side=Left
  N : Outport
  Ff : Outport  Port=2
  wires:
  PS-Simulink Converter4/1 -> Product/2  "N"
  PS-Simulink Converter1/1 -> Product1/1, Product/1
  PS-Simulink Converter2/1 -> Product1/2  "Ff1"
  Product/1 -> N/1
  Product1/1 -> Ff/1
  connections:
  Spatial Contact Force/LConn1 -- Point/RConn1
  PS-Simulink Converter1/LConn1 -- Spatial Contact Force/RConn2
  PS-Simulink Converter4/LConn1 -- Spatial Contact Force/RConn3
  Conn1/RConn1 -- Spatial Contact Force/RConn1
  Point/LConn1 -- Conn2/RConn1
  PS-Simulink Converter2/LConn1 -- Spatial Contact Force/RConn4

== system siglearmV7XYZforcecontrol/Lefet Robot/Left/Subsystem1 ==
  PS-Simulink Converter1 : nesl_utility/PS-Simulink Converter  PhysicalDomain=network_engine_domain  SubClassName=ps_output  LeftPortType=input  RightPortType=output  PseudoPeriodic=off  Frequencies=[]  VectorFormat=inherit  Unit=inherit  AffineConversion=off
  PS-Simulink Converter2 : nesl_utility/PS-Simulink Converter  PhysicalDomain=network_engine_domain  SubClassName=ps_output  LeftPortType=input  RightPortType=output  PseudoPeriodic=off  Frequencies=[]  VectorFormat=inherit  Unit=inherit  AffineConversion=off
  PS-Simulink Converter4 : nesl_utility/PS-Simulink Converter  PhysicalDomain=network_engine_domain  SubClassName=ps_output  LeftPortType=input  RightPortType=output  PseudoPeriodic=off  Frequencies=[]  VectorFormat=inherit  Unit=inherit  AffineConversion=off
  Point : sm_lib/Curves and Surfaces/Point  GraphicType=None  MarkerShape=Sphere  MarkerSize=10  GraphicVisPropType=SimpleVisualProperties  GraphicDiffuseColor=[0.5 0.5 0.5]  GraphicOpacity=1.0  GraphicSpecularColor=[0.5 0.5 0.5 1.0]  GraphicAmbientColor=[0.15 0.15 0.15 1.0]  GraphicEmissiveColor=[0.0 0.0 0.0 1.0]  GraphicShininess=75
  Product : Product
  Product1 : Product
  Spatial Contact Force : sm_lib/Forces and Torques/Spatial Contact Force  NormalForceType=SmoothSpringDamper  NormalStiffness=1e6  NormalStiffnessUnits=N/m  NormalDamping=1e3  NormalDampingUnits=N/(m/s)  NormalTransitionRegionWidth=1e-3  NormalTransitionRegionWidthUnits=m  FrictionType=SmoothStickSlip  CoefficientOfStaticFriction=0.5  CoefficientOfDynamicFriction=0.3  FrictionalCriticalVelocity=1e-3  FrictionalCriticalVelocityUnits=m/s  SenseContactSignal=on  SensePenetrationDepth=off  SenseSeparationDistance=off  SenseNormalForceMagnitude=on  SenseFrictionalForceMagnitude=on  SenseNormalVelocity=off  SenseTangentialVelocity=off  SenseContactBaseRotation=off  SenseContactBaseTranslation=off  SenseContactFollowerRotation=off  SenseContactFollowerTranslation=off  ZeroCrossDetectContactStartAndEnd=off
  Conn1 : PMIOPort  Side=Right
  Conn2 : PMIOPort  Port=2  Side=Left
  N : Outport
  Ff : Outport  Port=2
  wires:
  PS-Simulink Converter4/1 -> Product/2  "N"
  PS-Simulink Converter1/1 -> Product1/1, Product/1
  PS-Simulink Converter2/1 -> Product1/2  "Ff1"
  Product/1 -> N/1
  Product1/1 -> Ff/1
  connections:
  Spatial Contact Force/LConn1 -- Point/RConn1
  PS-Simulink Converter1/LConn1 -- Spatial Contact Force/RConn2
  PS-Simulink Converter4/LConn1 -- Spatial Contact Force/RConn3
  Conn1/RConn1 -- Spatial Contact Force/RConn1
  Point/LConn1 -- Conn2/RConn1
  PS-Simulink Converter2/LConn1 -- Spatial Contact Force/RConn4
